simulink subsystem "Environment"  (R2025b)
settings: Solver=VariableStepAuto  StartTime=0.0  StopTime=10.0  RelTol=1e-3
undefined symbols (not defined in the file): ln, Newton, Raphson, SimIn, SimPar
libraries: simulink x7, libAxisTransformations x1
settings Model: Creator=tbritton  LastModifiedBy=bullo
settings SolverCC: AlgebraicLoopSolver=TrustRegion
settings OptimizationCC: ReuseModelBlockBuffer=off
settings DebuggingCC: UnconnectedInputMsg=warning  UnconnectedOutputMsg=warning  UnconnectedLineMsg=warning
settings ModelReferenceCC: EnableRefExpFcnMdlSchedulingChecks=on
settings RTWCC: GPUComputeCapability=3.5  DLArmComputeVersion=19.05

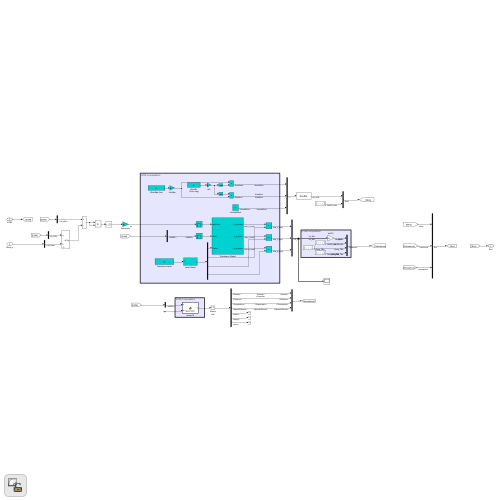
[thumbnail: Simulink's stored preview of the top-level diagram]
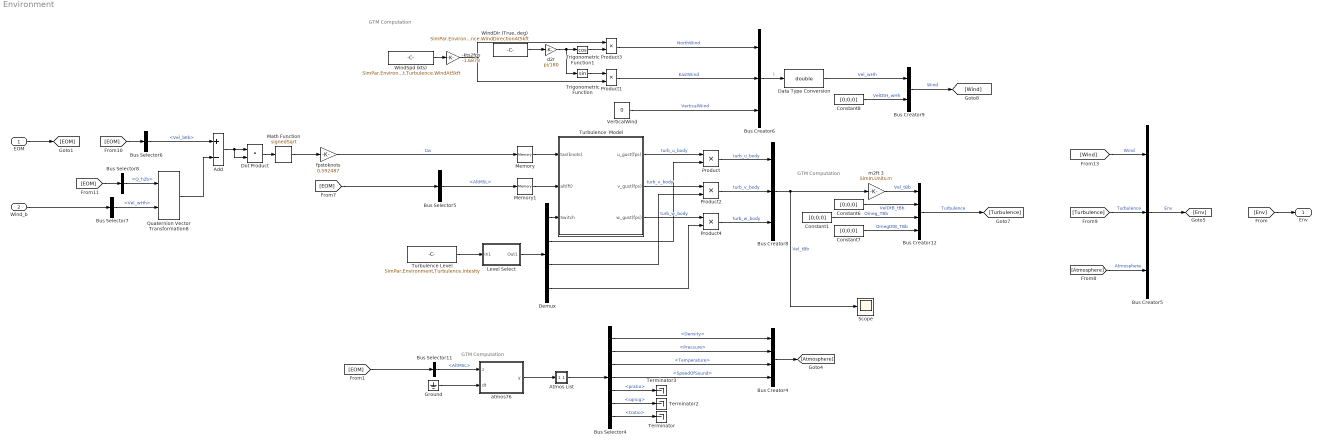
== system Environment ==
  note: GTM Computation
  note: GTM Computation
  note: GTM Computation
  EOM : Inport  OutDataTypeStr=Bus: EomBus
  Wind_b : Inport  Port=2
  -kts2fps : Gain  Gain=-1.6878  SaturateOnIntegerOverflow=on  OutDataTypeStr=Inherit: Same as input  ParamDataTypeStr=Inherit: Same as input
  Add : Sum  Inputs=+-
  Atmos List : Subsystem
  Bus Creator12 : BusCreator  Inputs=4  OutDataTypeStr=Bus: TurbulenceBus
  Bus Creator4 : BusCreator  Inputs=4
  Bus Creator5 : BusCreator  Inputs=3  OutDataTypeStr=Bus: EnvironmentBus
  Bus Creator6 : BusCreator  Inputs=3
  Bus Creator8 : BusCreator  Inputs=3
  Bus Creator9 : BusCreator  Inputs=2  OutDataTypeStr=Bus: WindBus
  Bus Selector11 : BusSelector  OutputSignals=WorldRelativeData.AltMSL
  Bus Selector4 : BusSelector  OutputSignals=Density,Pressure,Temperature,SpeedOfSound,pratio,sqrsig,tratio
  Bus Selector5 : BusSelector  OutputSignals=WorldRelativeData.AltMSL
  Bus Selector6 : BusSelector  OutputSignals=WorldRelativeData.Vel_bEb
  Bus Selector7 : BusSelector  OutputSignals=Wind.Vel_wHh
  Bus Selector8 : BusSelector  OutputSignals=WorldRelativeData.Q_h2b
  Constant{1,6..8} (4 alike) : Constant  Value=[0;0;0]
  Data Type Conversion : DataTypeConversion  OutDataTypeStr=double  SaturateOnIntegerOverflow=off  RndMeth=Floor
  Demux : Demux
  Dot Product : DotProduct  OutDataTypeStr=Inherit: Inherit via internal rule
  Ground : Ground
  Level Select : Subsystem
  Math Function : Sqrt  Operator=signedSqrt  AlgorithmType=Newton-Raphson
  Memory : Memory  InitialCondition=70
  Memory1 : Memory  InitialCondition=1000
  Product : Product  RndMeth=Zero
  Product1 : Product  Inputs=**  InputSameDT=on  SaturateOnIntegerOverflow=on  OutDataTypeStr=Inherit: Same as first input
  Product2 : Product  RndMeth=Zero
  Product3 : Product  Inputs=**  InputSameDT=on  SaturateOnIntegerOverflow=on  OutDataTypeStr=Inherit: Same as first input
  Product4 : Product  RndMeth=Zero
  Quaternion Vector Transformation8 : libAxisTransformations/Quaternion Vector Transformation  n=0
  Scope : Scope
      settings: DataLoggingVariableName=ScopeData16
  Terminator : Terminator
  Terminator2 : Terminator
  Terminator3 : Terminator
  Trigonometric Function : Trigonometry
  Trigonometric Function1 : Trigonometry  Operator=cos
  Turbulence  Model : Subsystem
  Turbulence Level : Constant  Value=SimPar.Environment.Turbulence.intesity
  VerticalWind : Constant  Value=0
  "WindDir (True, deg)" : Constant  Value=SimPar.Environment.Turbulence.WindDirectionAt5kft
  WindSpd (kts) : Constant  Value=SimPar.Environment.Turbulence.WindAt5kft
  atmos76 : MATLAB Function  TreatAsAtomicUnit=on
  d2r : Gain  Gain=pi/180  SaturateOnIntegerOverflow=on  OutDataTypeStr=Inherit: Same as input  ParamDataTypeStr=Inherit: Same as input
  fpstoknots : Gain  Gain=0.592487
  m2ft 3 : Gain  Gain=SimIn.Units.m
  Env : Outport  OutDataTypeStr=Bus: EnvironmentBus  VectorParamsAs1DForOutWhenUnconnected=off
  wires:
  Data Type Conversion/1 -> Bus Creator9/1  "Vel_wHh"
  [EOM] -> Bus Selector8/1
  [EOM] -> Bus Selector6/1
  Quaternion Vector Transformation8/1 -> Add/2
  fpstoknots/1 -> Memory/1  "tas"
  Math Function/1 -> fpstoknots/1
  Wind_b/1 -> Bus Selector7/1
  Add/1 -> Dot Product/1, Dot Product/2
  Dot Product/1 -> Math Function/1
  Bus Creator12/1 -> [Turbulence]  "Turbulence"
  Constant7/1 -> Bus Creator12/4  "OmegDtB_TBb"
  Constant6/1 -> Bus Creator12/2  "VelDtB_tBb"
  m2ft 3/1 -> Bus Creator12/1  "Vel_tBb"
  Constant1/1 -> Bus Creator12/3  "Omeg_TBb"
  [EOM] -> Bus Selector11/1
  Ground/1 -> atmos76/2(dt)
  Bus Selector11/1 -> atmos76/1(z)  "<AltMSL>"
  atmos76/1(y) -> Atmos List/1(I)
  Turbulence  Model/3(w_gust(fps)) -> Product4/1  "turb_w_body"
  Memory/1 -> Turbulence  Model/1(tas(knots))
  Level Select/1(Out1) -> Demux/1
  Turbulence  Model/1(u_gust(fps)) -> Product/1  "turb_u_body"
  Turbulence Level/1 -> Level Select/1(In1)
  Trigonometric Function/1 -> Product1/1
  Turbulence  Model/2(v_gust(fps)) -> Product2/1  "turb_v_body"
  "WindDir (True, deg)"/1 -> d2r/1
  d2r/1 -> Trigonometric Function/1, Trigonometric Function1/1
  Demux/1 -> Turbulence  Model/3(Switch)
  Demux/2 -> Product/2
  -kts2fps/1 -> Product3/1, Product1/2
  Demux/4 -> Product4/2
  Demux/3 -> Product2/2
  WindSpd (kts)/1 -> -kts2fps/1
  Trigonometric Function1/1 -> Product3/2
  Memory1/1 -> Turbulence  Model/2(alt(ft))
  [EOM] -> Bus Selector5/1
  Bus Selector5/1 -> Memory1/1  "<AltMSL>"
  [Turbulence] -> Bus Creator5/2  "Turbulence"
  [Wind] -> Bus Creator5/1  "Wind"
  [Atmosphere] -> Bus Creator5/3  "Atmosphere"
  Bus Creator5/1 -> [Env]  "Env"
  Bus Selector4/7 -> Terminator/1  "<tratio>"
  Bus Selector4/6 -> Terminator2/1  "<sqrsig>"
  Bus Selector4/5 -> Terminator3/1  "<pratio>"
  Atmos List/1(O) -> Bus Selector4/1
  [Env] -> Env/1
  EOM/1 -> [EOM]
  Bus Creator4/1 -> [Atmosphere]
  Bus Selector4/3 -> Bus Creator4/3  "<Temperature>"
  Bus Selector4/1 -> Bus Creator4/1  "<Density>"
  Bus Selector4/4 -> Bus Creator4/4  "<SpeedOfSound>"
  Bus Selector4/2 -> Bus Creator4/2  "<Pressure>"
  Product/1 -> Bus Creator8/1  "turb_u_body"
  Product2/1 -> Bus Creator8/2  "turb_v_body"
  Product4/1 -> Bus Creator8/3  "turb_w_body"
  Bus Selector6/1 -> Add/1  "<Vel_bEb>"
  Bus Selector8/1 -> Quaternion Vector Transformation8/1  "<Q_h2b>"
  Bus Selector7/1 -> Quaternion Vector Transformation8/2  "<Vel_wHh>"
  Constant8/1 -> Bus Creator9/2  "VelDtH_wHh"
  Product3/1 -> Bus Creator6/1  "NorthWind"
  Product1/1 -> Bus Creator6/2  "EastWind"
  Bus Creator9/1 -> [Wind]  "Wind"
  VerticalWind/1 -> Bus Creator6/3  "VerticalWind"
  Bus Creator6/1 -> Data Type Conversion/1  "l"
  Bus Creator8/1 -> Scope/1, m2ft 3/1  "Vel_tBb"

== system Environment/Atmos List ==
  I : Inport
  BusCreator : BusCreator  Inputs=7
  Demux2 : Demux  Outputs=6
      settings: DisplayOption=none
  Divide : Product  Inputs=*/
  Standard Temp. K : Constant  Value=288.15
  O : Outport  VectorParamsAs1DForOutWhenUnconnected=off
  wires:
  Demux2/6 -> BusCreator/6  "sqrsig"
  Demux2/5 -> BusCreator/5  "pratio"
  Demux2/4 -> BusCreator/4  "SpeedOfSound"
  Demux2/3 -> BusCreator/3, Divide/1  "Temperature"
  Demux2/2 -> BusCreator/2  "Pressure"
  Demux2/1 -> BusCreator/1  "Density"
  I/1 -> Demux2/1
  BusCreator/1 -> O/1
  Standard Temp. K/1 -> Divide/2
  Divide/1 -> BusCreator/7  "tratio"

== system Environment/Level Select ==
  In1 : Inport
  Light : Constant  Value=[1 0.2 0.2 0.17]
  Moderate : Constant  Value=[1 0.4 0.4 0.34]
  Multiport Switch : MultiPortSwitch  Inputs=4  SaturateOnIntegerOverflow=off  InputSameDT=off
  Severe : Constant  Value=[1 0.4 1.152 0.34]
  Turbulence Off : Constant  Value=[0 0 0 0]
  Out1 : Outport
  wires:
  In1/1 -> Multiport Switch/1
  Turbulence Off/1 -> Multiport Switch/2
  Light/1 -> Multiport Switch/3
  Moderate/1 -> Multiport Switch/4
  Severe/1 -> Multiport Switch/5
  Multiport Switch/1 -> Out1/1

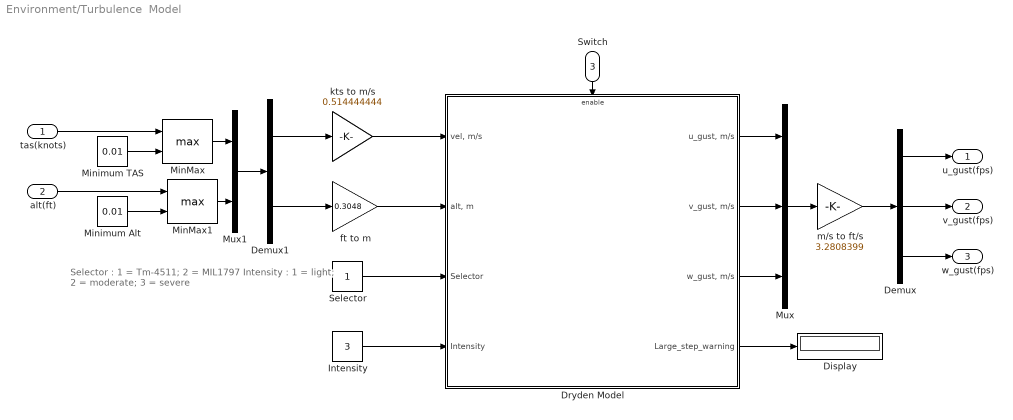
== system Environment/Turbulence  Model ==
  note: Selector :  1 = Tm-4511;  2 = MIL1797
      |             Intensity :  1 = light;  2 = moderate;  3 = severe
  tas(knots) : Inport
  alt(ft) : Inport  Port=2
  Switch : Inport  Port=3
  Demux : Demux  Outputs=3
  Demux1 : Demux  Outputs=2
  Display : Display
  Dryden Model : Subsystem  mask{longseed=3366+521, latseed=23+521, vertseed=1369+521, dt=SimIn.Environment.Turbulence.dT, Step_warning_pct=.11}
      mask prompts: longseed "Longitudinal Random Number Seed"; latseed "Lateral Random Number Seed"; vertseed "Vertical Random Number Seed"; dt "Turbulence model time step, sec"; Step_warning_pct "Threshhold for stepsize warning (%)"
  Intensity : Constant  Value=3
  MinMax : MinMax  Function=max  Inputs=2
  MinMax1 : MinMax  Function=max  Inputs=2
  Minimum Alt : Constant  Value=0.01
  Minimum TAS : Constant  Value=0.01
  Mux : Mux  Inputs=3
  Mux1 : Mux  Inputs=2
  Selector : Constant
  ft to m : Gain  Gain=0.3048
  kts to m/s : Gain  Gain=0.514444444
  m/s to ft/s : Gain  Gain=3.2808399
  u_gust(fps) : Outport
  v_gust(fps) : Outport  Port=2
  w_gust(fps) : Outport  Port=3
  wires:
  Switch/1 -> Dryden Model/Enable
  Dryden Model/1("u_gust, m/s") -> Mux/1
  Dryden Model/2("v_gust, m/s") -> Mux/2
  Dryden Model/3("w_gust, m/s") -> Mux/3
  Demux/3 -> w_gust(fps)/1
  Demux/2 -> v_gust(fps)/1
  Demux/1 -> u_gust(fps)/1
  Dryden Model/4(Large_step_warning) -> Display/1
  Mux/1 -> m/s to ft/s/1
  m/s to ft/s/1 -> Demux/1
  MinMax1/1 -> Mux1/2
  MinMax/1 -> Mux1/1
  alt(ft)/1 -> MinMax1/1
  Minimum Alt/1 -> MinMax1/2
  Minimum TAS/1 -> MinMax/2
  tas(knots)/1 -> MinMax/1
  Mux1/1 -> Demux1/1
  Demux1/2 -> ft to m/1
  Demux1/1 -> kts to m/s/1
  Intensity/1 -> Dryden Model/4(Intensity)
  Selector/1 -> Dryden Model/3(Selector)
  ft to m/1 -> Dryden Model/2("alt, m")
  kts to m/s/1 -> Dryden Model/1("vel, m/s")

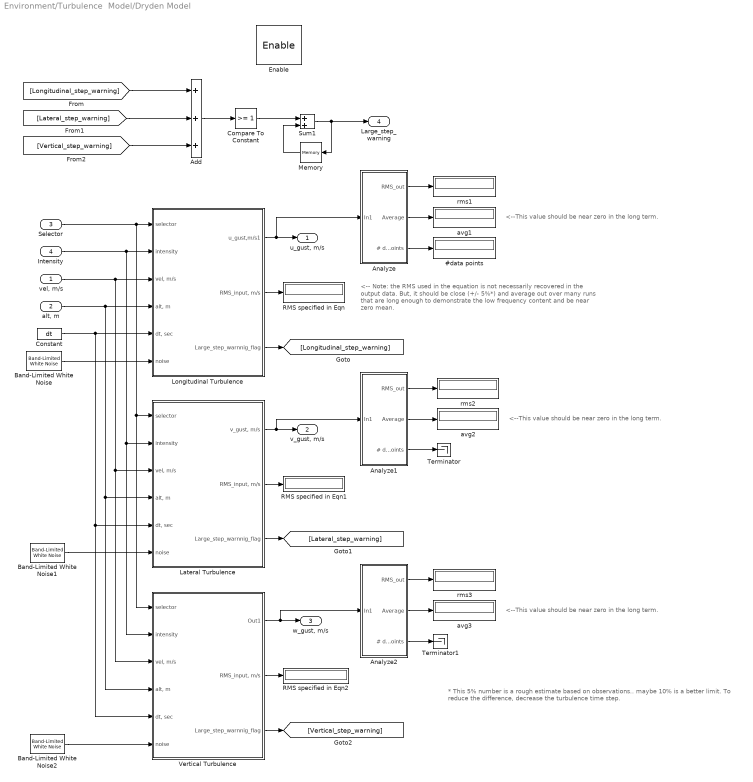
== system Environment/Turbulence  Model/Dryden Model ==
  note: * This 5% number is a rough estimate based on observations.. maybe 10% is a better limit.
      | To reduce the difference, decrease the turbulence time step.
  note: <--This value should be near zero in the long term.
  note: <--This value should be near zero in the long term.
  note: <--This value should be near zero in the long term.
  note: <-- Note: the RMS used in the equation is not necessarily recovered
      | in the output data.  But, it should be close (+/- 5%*) and  average out over
      | many runs that are long enough to demonstrate the low frequency
      | content and be near zero mean.
  "vel, m/s" : Inport
  "alt, m" : Inport  Port=2
  Selector : Inport  Port=3
  Intensity : Inport  Port=4
  Enable : EnablePort  StatesWhenEnabling=reset
  #data points : Display
  Add : Sum  Inputs=3
  Analyze : Subsystem
  Analyze1 : Subsystem
  Analyze2 : Subsystem
  Band-Limited White Noise : simulink/Sources/Band-Limited White Noise  Cov=dt  Ts=dt  seed=longseed
  Band-Limited White Noise1 : simulink/Sources/Band-Limited White Noise  Cov=dt  Ts=dt  seed=latseed
  Band-Limited White Noise2 : simulink/Sources/Band-Limited White Noise  Cov=dt  Ts=dt  seed=vertseed
  Compare To Constant : simulink/Logic and Bit Operations/Compare To Constant  relop=>=  const=1  OutDataTypeStr=uint8  ZeroCross=off
  Constant : Constant  Value=dt
  Lateral Turbulence : Subsystem
  Longitudinal Turbulence : Subsystem
  Memory : Memory
  RMS specified in Eqn : Display
  RMS specified in Eqn1 : Display
  RMS specified in Eqn2 : Display
  Sum1 : Sum  Inputs=2  SaturateOnIntegerOverflow=on
  Terminator : Terminator
  Terminator1 : Terminator
  Vertical Turbulence : Subsystem
  avg1 : Display
  avg2 : Display
  avg3 : Display
  rms1 : Display
  rms2 : Display
  rms3 : Display
  "u_gust, m/s" : Outport  OutputWhenDisabled=reset  InitialOutput=0
  "v_gust, m/s" : Outport  Port=2  OutputWhenDisabled=reset  InitialOutput=0
  "w_gust, m/s" : Outport  Port=3  OutputWhenDisabled=reset  InitialOutput=0
  Large_step_warning : Outport  Port=4  OutputWhenDisabled=reset  InitialOutput=0
  wires:
  Sum1/1 -> Memory/1, Large_step_warning/1
  Memory/1 -> Sum1/2
  Compare To Constant/1 -> Sum1/1
  Vertical Turbulence/3(Large_step_warnnig_flag) -> [Vertical_step_warning]
  Lateral Turbulence/3(Large_step_warnnig_flag) -> [Lateral_step_warning]
  Longitudinal Turbulence/3(Large_step_warnnig_flag) -> [Longitudinal_step_warning]
  [Lateral_step_warning] -> Add/2
  [Vertical_step_warning] -> Add/3
  [Longitudinal_step_warning] -> Add/1
  Add/1 -> Compare To Constant/1
  Band-Limited White Noise/1 -> Longitudinal Turbulence/6(noise)
  Analyze2/3(# data points) -> Terminator1/1
  Analyze1/3(# data points) -> Terminator/1
  Analyze/3(# data points) -> #data points/1
  Vertical Turbulence/2("RMS_input, m/s") -> RMS specified in Eqn2/1
  Lateral Turbulence/2("RMS_input, m/s") -> RMS specified in Eqn1/1
  Longitudinal Turbulence/2("RMS_input, m/s") -> RMS specified in Eqn/1
  Analyze2/2(Average) -> avg3/1
  Analyze2/1(RMS_out) -> rms3/1
  Vertical Turbulence/1(Out1) -> Analyze2/1(In1), "w_gust, m/s"/1
  Analyze1/2(Average) -> avg2/1
  Analyze1/1(RMS_out) -> rms2/1
  Lateral Turbulence/1("v_gust, m/s") -> Analyze1/1(In1), "v_gust, m/s"/1
  Analyze/2(Average) -> avg1/1
  Longitudinal Turbulence/1(u_gust,m/s1) -> Analyze/1(In1), "u_gust, m/s"/1
  Analyze/1(RMS_out) -> rms1/1
  Intensity/1 -> Lateral Turbulence/2(intensity), Vertical Turbulence/2(intensity), Longitudinal Turbulence/2(intensity)
  Band-Limited White Noise2/1 -> Vertical Turbulence/6(noise)
  Selector/1 -> Lateral Turbulence/1(selector), Vertical Turbulence/1(selector), Longitudinal Turbulence/1(selector)
  Band-Limited White Noise1/1 -> Lateral Turbulence/6(noise)
  Constant/1 -> Lateral Turbulence/5("dt, sec"), Vertical Turbulence/5("dt, sec"), Longitudinal Turbulence/5("dt, sec")
  "alt, m"/1 -> Lateral Turbulence/4("alt, m"), Vertical Turbulence/4("alt, m"), Longitudinal Turbulence/4("alt, m")
  "vel, m/s"/1 -> Lateral Turbulence/3("vel, m/s"), Vertical Turbulence/3("vel, m/s"), Longitudinal Turbulence/3("vel, m/s")

== system Environment/Turbulence  Model/Dryden Model/Analyze ==
  In1 : Inport
  Constant1 : Constant
  Constant3 : Constant  Value=0
  Constant5 : Constant  Value=dt
  Digital Clock1 : DigitalClock  SampleTime=dt
  Fcn : Fcn  Expr=sqrt(u)
  Memory : Memory
  Memory1 : Memory
  MinMax : MinMax  Function=max  Inputs=2
  Product : Product  SaturateOnIntegerOverflow=on  OutDataTypeStr=Inherit: Same as first input
  Product2 : Product  Inputs=/*  SaturateOnIntegerOverflow=on  OutDataTypeStr=Inherit: Same as first input
  Product3 : Product  Inputs=/*  SaturateOnIntegerOverflow=on  OutDataTypeStr=Inherit: Same as first input
  Product4 : Product  Inputs=/*  SaturateOnIntegerOverflow=on  OutDataTypeStr=Inherit: Same as first input
  Sum : Sum  Inputs=++-  SaturateOnIntegerOverflow=on
  Sum1 : Sum  Inputs=2  SaturateOnIntegerOverflow=on
  RMS_out : Outport
  Average : Outport  Port=2
  # data points : Outport  Port=3
  wires:
  MinMax/1 -> Product2/1, Product4/1
  Constant1/1 -> MinMax/2
  In1/1 -> Sum1/1, Product/1, Product/2
  Product/1 -> Sum/2
  Sum/1 -> Memory1/1, Product2/2
  Sum1/1 -> Memory/1, Product4/2
  Product2/1 -> Fcn/1
  Memory/1 -> Sum1/2
  Memory1/1 -> Sum/1
  Constant3/1 -> Sum/3
  Constant5/1 -> Product3/1
  Digital Clock1/1 -> Product3/2
  Product3/1 -> MinMax/1, # data points/1
  Fcn/1 -> RMS_out/1
  Product4/1 -> Average/1

== system Environment/Turbulence  Model/Dryden Model/Analyze1 ==
  In1 : Inport
  Constant1 : Constant
  Constant3 : Constant  Value=0
  Constant5 : Constant  Value=dt
  Digital Clock1 : DigitalClock  SampleTime=dt
  Fcn : Fcn  Expr=sqrt(u)
  Memory : Memory
  Memory1 : Memory
  MinMax : MinMax  Function=max  Inputs=2
  Product : Product  SaturateOnIntegerOverflow=on  OutDataTypeStr=Inherit: Same as first input
  Product2 : Product  Inputs=/*  SaturateOnIntegerOverflow=on  OutDataTypeStr=Inherit: Same as first input
  Product3 : Product  Inputs=/*  SaturateOnIntegerOverflow=on  OutDataTypeStr=Inherit: Same as first input
  Product4 : Product  Inputs=/*  SaturateOnIntegerOverflow=on  OutDataTypeStr=Inherit: Same as first input
  Sum : Sum  Inputs=++-  SaturateOnIntegerOverflow=on
  Sum1 : Sum  Inputs=2  SaturateOnIntegerOverflow=on
  RMS_out : Outport
  Average : Outport  Port=2
  # data points : Outport  Port=3
  wires:
  Product4/1 -> Average/1
  Fcn/1 -> RMS_out/1
  Product3/1 -> # data points/1, MinMax/1
  Digital Clock1/1 -> Product3/2
  Constant5/1 -> Product3/1
  Constant3/1 -> Sum/3
  Memory1/1 -> Sum/1
  Memory/1 -> Sum1/2
  Product2/1 -> Fcn/1
  Sum1/1 -> Product4/2, Memory/1
  Sum/1 -> Product2/2, Memory1/1
  Product/1 -> Sum/2
  In1/1 -> Product/2, Product/1, Sum1/1
  Constant1/1 -> MinMax/2
  MinMax/1 -> Product4/1, Product2/1

== system Environment/Turbulence  Model/Dryden Model/Analyze2 ==
  In1 : Inport
  Constant1 : Constant
  Constant3 : Constant  Value=0
  Constant5 : Constant  Value=dt
  Digital Clock1 : DigitalClock  SampleTime=dt
  Fcn : Fcn  Expr=sqrt(u)
  Memory : Memory
  Memory1 : Memory
  MinMax : MinMax  Function=max  Inputs=2
  Product : Product  SaturateOnIntegerOverflow=on  OutDataTypeStr=Inherit: Same as first input
  Product2 : Product  Inputs=/*  SaturateOnIntegerOverflow=on  OutDataTypeStr=Inherit: Same as first input
  Product3 : Product  Inputs=/*  SaturateOnIntegerOverflow=on  OutDataTypeStr=Inherit: Same as first input
  Product4 : Product  Inputs=/*  SaturateOnIntegerOverflow=on  OutDataTypeStr=Inherit: Same as first input
  Sum : Sum  Inputs=++-  SaturateOnIntegerOverflow=on
  Sum1 : Sum  Inputs=2  SaturateOnIntegerOverflow=on
  RMS_out : Outport
  Average : Outport  Port=2
  # data points : Outport  Port=3
  wires:
  MinMax/1 -> Product2/1, Product4/1
  Constant1/1 -> MinMax/2
  In1/1 -> Sum1/1, Product/1, Product/2
  Product/1 -> Sum/2
  Sum/1 -> Memory1/1, Product2/2
  Sum1/1 -> Memory/1, Product4/2
  Product2/1 -> Fcn/1
  Memory/1 -> Sum1/2
  Memory1/1 -> Sum/1
  Constant3/1 -> Sum/3
  Constant5/1 -> Product3/1
  Digital Clock1/1 -> Product3/2
  Product3/1 -> MinMax/1, # data points/1
  Fcn/1 -> RMS_out/1
  Product4/1 -> Average/1

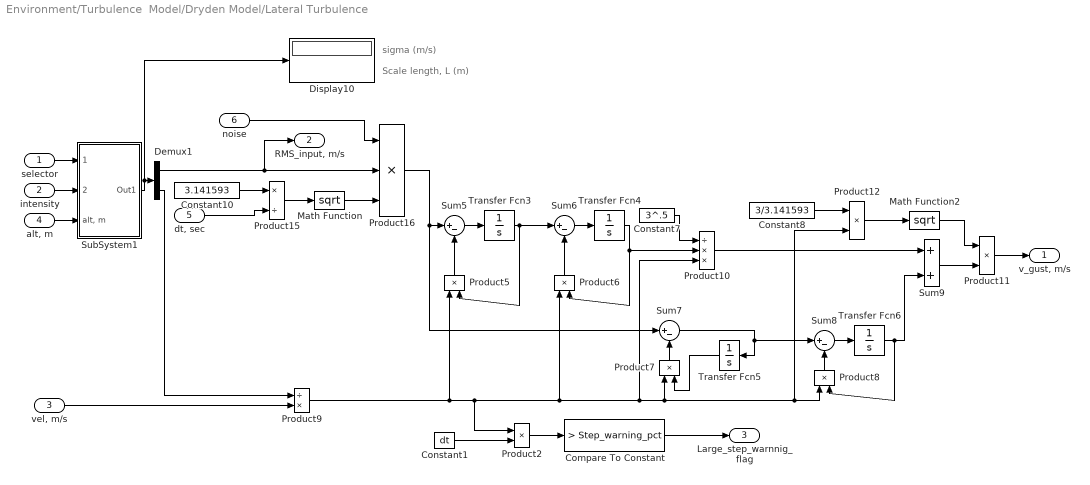
== system Environment/Turbulence  Model/Dryden Model/Lateral Turbulence ==
  note: Scale length, L (m)
  note: sigma (m/s)
  selector : Inport
  intensity : Inport  Port=2
  "vel, m/s" : Inport  Port=3
  "alt, m" : Inport  Port=4
  "dt, sec" : Inport  Port=5
  noise : Inport  Port=6
  Compare To Constant : simulink/Logic and Bit Operations/Compare To Constant  relop=>  const=Step_warning_pct  OutDataTypeStr=uint8  ZeroCross=off
  Constant1 : Constant  Value=dt
  Constant10 : Constant  Value=3.141593
  Constant7 : Constant  Value=3^.5
  Constant8 : Constant  Value=3/3.141593
  Demux1 : Demux  Outputs=2
      settings: DisplayOption=none
  Display10 : Display
  Math Function : Math  Operator=sqrt  SignedPower=on
  Math Function2 : Math  Operator=sqrt  SignedPower=on
  Product10 : Product  Inputs=/**  InputSameDT=on  SaturateOnIntegerOverflow=on  OutDataTypeStr=Inherit: Same as first input
  Product11 : Product  Inputs=**  InputSameDT=on  SaturateOnIntegerOverflow=on  OutDataTypeStr=Inherit: Same as first input
  Product12 : Product  Inputs=**  InputSameDT=on  SaturateOnIntegerOverflow=on  OutDataTypeStr=Inherit: Same as first input
  Product15 : Product  Inputs=*/  InputSameDT=on  SaturateOnIntegerOverflow=on  OutDataTypeStr=Inherit: Same as first input
  Product16 : Product  Inputs=***  InputSameDT=on  SaturateOnIntegerOverflow=on  OutDataTypeStr=Inherit: Same as first input
  Product{2,5..8} (5 alike) : Product  InputSameDT=on  SaturateOnIntegerOverflow=on  OutDataTypeStr=Inherit: Same as first input
  Product9 : Product  Inputs=/*  InputSameDT=on  SaturateOnIntegerOverflow=on  OutDataTypeStr=Inherit: Same as first input
  SubSystem1 : Subsystem
  Sum{5..8} (4 alike) : Sum  Inputs=|+-  InputSameDT=on  SaturateOnIntegerOverflow=on  OutDataTypeStr=Inherit: Same as first input
  Sum9 : Sum  Inputs=2  InputSameDT=on  SaturateOnIntegerOverflow=on  OutDataTypeStr=Inherit: Same as first input
  Transfer Fcn{3..6} (4 alike) : TransferFcn  Numerator=1  Denominator=[1 0]
  "v_gust, m/s" : Outport
  "RMS_input, m/s" : Outport  Port=2
  Large_step_warnnig_flag : Outport  Port=3
  wires:
  Compare To Constant/1 -> Large_step_warnnig_flag/1
  Product2/1 -> Compare To Constant/1
  Constant1/1 -> Product2/2
  Math Function/1 -> Product16/3
  intensity/1 -> SubSystem1/2(intensity)
  selector/1 -> SubSystem1/1(selector)
  "alt, m"/1 -> SubSystem1/3("alt, m")
  Demux1/2 -> Product9/1
  SubSystem1/1(Out1) -> Display10/1, Demux1/1
  Product16/1 -> Sum7/1, Sum5/1
  Demux1/1 -> Product16/2, "RMS_input, m/s"/1
  "dt, sec"/1 -> Product15/2
  Product9/1 -> Product2/1, Product10/3, Product12/2, Product8/1, Product7/1, Product6/1, Product5/1
  "vel, m/s"/1 -> Product9/2
  Product12/1 -> Math Function2/1
  Constant8/1 -> Product12/1
  Math Function2/1 -> Product11/1
  Sum9/1 -> Product11/2
  Constant7/1 -> Product10/1
  Product10/1 -> Sum9/1
  Transfer Fcn6/1 -> Sum9/2, Product8/2
  Sum7/1 -> Sum8/1, Transfer Fcn5/1
  Product8/1 -> Sum8/2
  Sum8/1 -> Transfer Fcn6/1
  Product7/1 -> Sum7/2
  Transfer Fcn5/1 -> Product7/2
  Transfer Fcn4/1 -> Product10/2, Product6/2
  Transfer Fcn3/1 -> Sum6/1, Product5/2
  Product6/1 -> Sum6/2
  Sum6/1 -> Transfer Fcn4/1
  Sum5/1 -> Transfer Fcn3/1
  Product5/1 -> Sum5/2
  noise/1 -> Product16/1
  Constant10/1 -> Product15/1
  Product15/1 -> Math Function/1
  Product11/1 -> "v_gust, m/s"/1

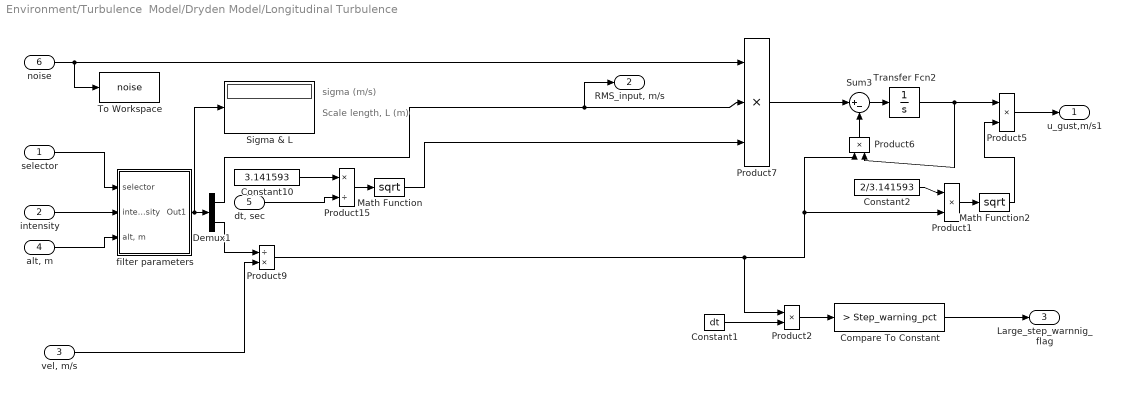
== system Environment/Turbulence  Model/Dryden Model/Longitudinal Turbulence ==
  note: Scale length, L (m)
  note: sigma (m/s)
  selector : Inport
  intensity : Inport  Port=2
  "vel, m/s" : Inport  Port=3
  "alt, m" : Inport  Port=4
  "dt, sec" : Inport  Port=5
  noise : Inport  Port=6
  Compare To Constant : simulink/Logic and Bit Operations/Compare To Constant  relop=>  const=Step_warning_pct  OutDataTypeStr=uint8  ZeroCross=off
  Constant1 : Constant  Value=dt
  Constant10 : Constant  Value=3.141593
  Constant2 : Constant  Value=2/3.141593
  Demux1 : Demux  Outputs=2
      settings: DisplayOption=none
  Math Function : Math  Operator=sqrt  SignedPower=on
  Math Function2 : Math  Operator=sqrt  SignedPower=on
  Product1 : Product  Inputs=**  InputSameDT=on  SaturateOnIntegerOverflow=on  OutDataTypeStr=Inherit: Same as first input
  Product15 : Product  Inputs=*/  InputSameDT=on  SaturateOnIntegerOverflow=on  OutDataTypeStr=Inherit: Same as first input
  Product2 : Product  InputSameDT=on  SaturateOnIntegerOverflow=on  OutDataTypeStr=Inherit: Same as first input
  Product5 : Product  Inputs=**  InputSameDT=on  SaturateOnIntegerOverflow=on  OutDataTypeStr=Inherit: Same as first input
  Product6 : Product  InputSameDT=on  SaturateOnIntegerOverflow=on  OutDataTypeStr=Inherit: Same as first input
  Product7 : Product  Inputs=***  InputSameDT=on  SaturateOnIntegerOverflow=on  OutDataTypeStr=Inherit: Same as first input
  Product9 : Product  Inputs=/*  InputSameDT=on  SaturateOnIntegerOverflow=on  OutDataTypeStr=Inherit: Same as first input
  Sigma & L : Display
  Sum3 : Sum  Inputs=|+-  InputSameDT=on  SaturateOnIntegerOverflow=on  OutDataTypeStr=Inherit: Same as first input
  To Workspace : ToWorkspace  VariableName=noise  SampleTime=-1
  Transfer Fcn2 : TransferFcn  Numerator=1  Denominator=[1 0]
  filter parameters : Subsystem
  u_gust,m/s1 : Outport
  "RMS_input, m/s" : Outport  Port=2
  Large_step_warnnig_flag : Outport  Port=3
  wires:
  Compare To Constant/1 -> Large_step_warnnig_flag/1
  Product2/1 -> Compare To Constant/1
  Constant1/1 -> Product2/2
  Product7/1 -> Sum3/1
  Product6/1 -> Sum3/2
  Product5/1 -> u_gust,m/s1/1
  Math Function2/1 -> Product5/2
  Product1/1 -> Math Function2/1
  Constant2/1 -> Product1/1
  Sum3/1 -> Transfer Fcn2/1
  Transfer Fcn2/1 -> Product5/1, Product6/2
  intensity/1 -> filter parameters/2(intensity)
  Demux1/1 -> "RMS_input, m/s"/1, Product7/2
  Demux1/2 -> Product9/1
  filter parameters/1(Out1) -> Demux1/1, Sigma & L/1
  noise/1 -> Product7/1, To Workspace/1
  "dt, sec"/1 -> Product15/2
  "vel, m/s"/1 -> Product9/2
  Constant10/1 -> Product15/1
  Product9/1 -> Product2/1, Product1/2, Product6/1
  Math Function/1 -> Product7/3
  Product15/1 -> Math Function/1
  selector/1 -> filter parameters/1(selector)
  "alt, m"/1 -> filter parameters/3("alt, m")

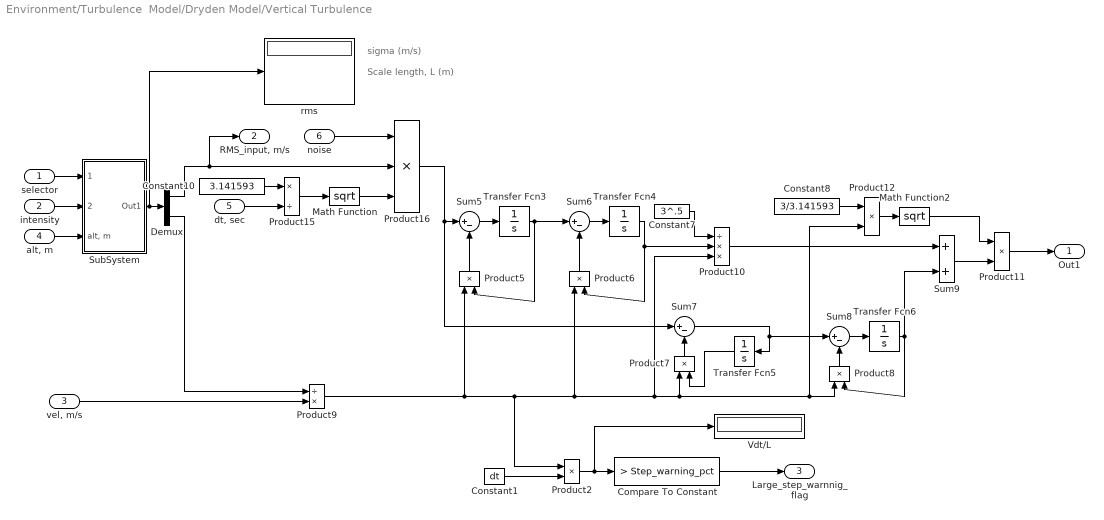
== system Environment/Turbulence  Model/Dryden Model/Vertical Turbulence ==
  note: Scale length, L (m)
  note: sigma (m/s)
  selector : Inport
  intensity : Inport  Port=2
  "vel, m/s" : Inport  Port=3
  "alt, m" : Inport  Port=4
  "dt, sec" : Inport  Port=5
  noise : Inport  Port=6
  Compare To Constant : simulink/Logic and Bit Operations/Compare To Constant  relop=>  const=Step_warning_pct  OutDataTypeStr=uint8  ZeroCross=off
  Constant1 : Constant  Value=dt
  Constant10 : Constant  Value=3.141593
  Constant7 : Constant  Value=3^.5
  Constant8 : Constant  Value=3/3.141593
  Demux : Demux  Outputs=2
      settings: DisplayOption=none
  Math Function : Math  Operator=sqrt  SignedPower=on
  Math Function2 : Math  Operator=sqrt  SignedPower=on
  Product10 : Product  Inputs=/**  InputSameDT=on  SaturateOnIntegerOverflow=on  OutDataTypeStr=Inherit: Same as first input
  Product11 : Product  Inputs=**  InputSameDT=on  SaturateOnIntegerOverflow=on  OutDataTypeStr=Inherit: Same as first input
  Product12 : Product  Inputs=**  InputSameDT=on  SaturateOnIntegerOverflow=on  OutDataTypeStr=Inherit: Same as first input
  Product15 : Product  Inputs=*/  InputSameDT=on  SaturateOnIntegerOverflow=on  OutDataTypeStr=Inherit: Same as first input
  Product16 : Product  Inputs=***  InputSameDT=on  SaturateOnIntegerOverflow=on  OutDataTypeStr=Inherit: Same as first input
  Product{2,5..8} (5 alike) : Product  InputSameDT=on  SaturateOnIntegerOverflow=on  OutDataTypeStr=Inherit: Same as first input
  Product9 : Product  Inputs=/*  InputSameDT=on  SaturateOnIntegerOverflow=on  OutDataTypeStr=Inherit: Same as first input
  SubSystem : Subsystem
  Sum{5..8} (4 alike) : Sum  Inputs=|+-  InputSameDT=on  SaturateOnIntegerOverflow=on  OutDataTypeStr=Inherit: Same as first input
  Sum9 : Sum  Inputs=2  InputSameDT=on  SaturateOnIntegerOverflow=on  OutDataTypeStr=Inherit: Same as first input
  Transfer Fcn{3..6} (4 alike) : TransferFcn  Numerator=1  Denominator=[1 0]
  Vdt/L : Display
  rms : Display
  Out1 : Outport
  "RMS_input, m/s" : Outport  Port=2
  Large_step_warnnig_flag : Outport  Port=3
  wires:
  Compare To Constant/1 -> Large_step_warnnig_flag/1
  Product2/1 -> Vdt/L/1, Compare To Constant/1
  Constant1/1 -> Product2/2
  intensity/1 -> SubSystem/2("intensity ")
  selector/1 -> SubSystem/1(selector)
  "alt, m"/1 -> SubSystem/3("alt, m")
  SubSystem/1(Out1) -> rms/1, Demux/1
  Demux/2 -> Product9/1
  Demux/1 -> "RMS_input, m/s"/1, Product16/2
  noise/1 -> Product16/1
  Product16/1 -> Sum7/1, Sum5/1
  "dt, sec"/1 -> Product15/2
  Math Function/1 -> Product16/3
  Product9/1 -> Product2/1, Product6/1, Product10/3, Product12/2, Product8/1, Product7/1, Product5/1
  "vel, m/s"/1 -> Product9/2
  Product12/1 -> Math Function2/1
  Constant8/1 -> Product12/1
  Math Function2/1 -> Product11/1
  Sum9/1 -> Product11/2
  Constant7/1 -> Product10/1
  Product10/1 -> Sum9/1
  Transfer Fcn6/1 -> Sum9/2, Product8/2
  Sum7/1 -> Sum8/1, Transfer Fcn5/1
  Product8/1 -> Sum8/2
  Sum8/1 -> Transfer Fcn6/1
  Product7/1 -> Sum7/2
  Transfer Fcn5/1 -> Product7/2
  Transfer Fcn4/1 -> Product10/2, Product6/2
  Transfer Fcn3/1 -> Sum6/1, Product5/2
  Product6/1 -> Sum6/2
  Sum6/1 -> Transfer Fcn4/1
  Sum5/1 -> Transfer Fcn3/1
  Product5/1 -> Sum5/2
  Constant10/1 -> Product15/1
  Product15/1 -> Math Function/1
  Product11/1 -> Out1/1

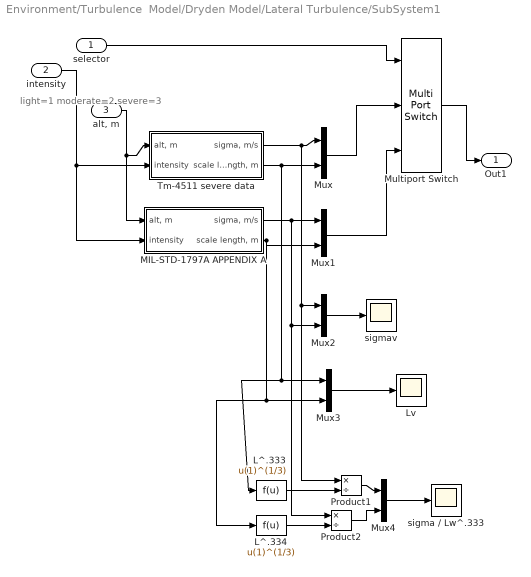
== system Environment/Turbulence  Model/Dryden Model/Lateral Turbulence/SubSystem1 ==
  note: light=1
      | moderate=2
      | severe=3
  selector : Inport
  intensity : Inport  Port=2
  "alt, m" : Inport  Port=3
  L^.333 : Fcn  Expr=u(1)^(1/3)
  L^.334 : Fcn  Expr=u(1)^(1/3)
  Lv : Scope
  "MIL-STD-1797A APPENDIX A " : Subsystem
  Multiport Switch : MultiPortSwitch  Inputs=2
  Mux{,1..4} (5 alike) : Mux  Inputs=2
  Product1 : Product  Inputs=*/  InputSameDT=on  SaturateOnIntegerOverflow=on  OutDataTypeStr=Inherit: Same as first input
  Product2 : Product  Inputs=*/  InputSameDT=on  SaturateOnIntegerOverflow=on  OutDataTypeStr=Inherit: Same as first input
  Tm-4511 severe data : Subsystem
  sigma / Lw^.333 : Scope
  sigmav : Scope
  Out1 : Outport
  wires:
  L^.333/1 -> Product1/2
  Product1/1 -> Mux4/1
  Product2/1 -> Mux4/2
  Mux4/1 -> sigma / Lw^.333/1
  L^.334/1 -> Product2/2
  "MIL-STD-1797A APPENDIX A "/2("scale length, m") -> L^.334/1, Mux3/2, Mux1/2
  Tm-4511 severe data/2("scale length, m") -> L^.333/1, Mux3/1, Mux/2
  "MIL-STD-1797A APPENDIX A "/1("sigma, m/s") -> Product2/1, Mux2/2, Mux1/1
  Mux2/1 -> sigmav/1
  Mux3/1 -> Lv/1
  Mux1/1 -> Multiport Switch/3
  intensity/1 -> Tm-4511 severe data/2(intensity), "MIL-STD-1797A APPENDIX A "/2(intensity)
  "alt, m"/1 -> "MIL-STD-1797A APPENDIX A "/1("alt, m"), Tm-4511 severe data/1("alt, m")
  Mux/1 -> Multiport Switch/2
  Tm-4511 severe data/1("sigma, m/s") -> Product1/1, Mux2/1, Mux/1
  Multiport Switch/1 -> Out1/1
  selector/1 -> Multiport Switch/1

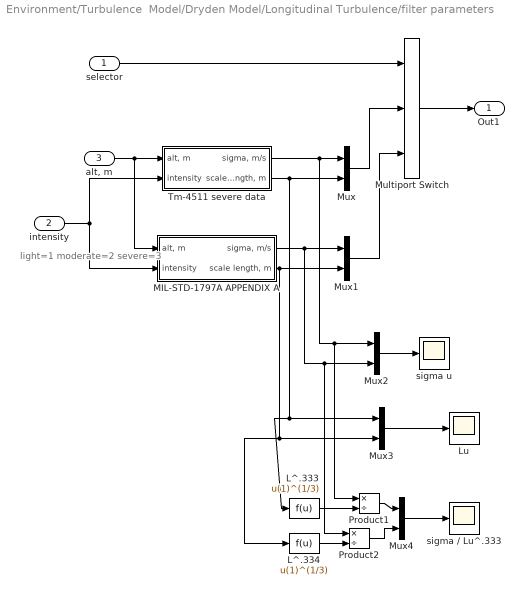
== system Environment/Turbulence  Model/Dryden Model/Longitudinal Turbulence/filter parameters ==
  note: light=1
      | moderate=2
      | severe=3
  selector : Inport
  intensity : Inport  Port=2
  "alt, m" : Inport  Port=3
  L^.333 : Fcn  Expr=u(1)^(1/3)
  L^.334 : Fcn  Expr=u(1)^(1/3)
  Lu : Scope
  "MIL-STD-1797A APPENDIX A " : Subsystem
  Multiport Switch : MultiPortSwitch  Inputs=2
  Mux{,1..4} (5 alike) : Mux  Inputs=2
  Product1 : Product  Inputs=*/  InputSameDT=on  SaturateOnIntegerOverflow=on  OutDataTypeStr=Inherit: Same as first input
  Product2 : Product  Inputs=*/  InputSameDT=on  SaturateOnIntegerOverflow=on  OutDataTypeStr=Inherit: Same as first input
  Tm-4511 severe data : Subsystem
  sigma / Lu^.333 : Scope
      settings: ActiveDisplayYMinimum=0  ActiveDisplayYMaximum=60
  sigma u : Scope
      settings: ActiveDisplayYMinimum=2  ActiveDisplayYMaximum=5.75
  Out1 : Outport
  wires:
  L^.334/1 -> Product2/2
  L^.333/1 -> Product1/2
  Product1/1 -> Mux4/1
  Product2/1 -> Mux4/2
  Mux4/1 -> sigma / Lu^.333/1
  "MIL-STD-1797A APPENDIX A "/2("scale length, m") -> L^.334/1, Mux3/2, Mux1/2
  Tm-4511 severe data/2("scale length, m") -> L^.333/1, Mux3/1, Mux/2
  "MIL-STD-1797A APPENDIX A "/1("sigma, m/s") -> Product2/1, Mux2/2, Mux1/1
  Mux2/1 -> sigma u/1
  Mux3/1 -> Lu/1
  intensity/1 -> Tm-4511 severe data/2(intensity), "MIL-STD-1797A APPENDIX A "/2(intensity)
  "alt, m"/1 -> "MIL-STD-1797A APPENDIX A "/1("alt, m"), Tm-4511 severe data/1("alt, m")
  Mux1/1 -> Multiport Switch/3
  Mux/1 -> Multiport Switch/2
  Tm-4511 severe data/1("sigma, m/s") -> Mux/1, Product1/1, Mux2/1
  Multiport Switch/1 -> Out1/1
  selector/1 -> Multiport Switch/1

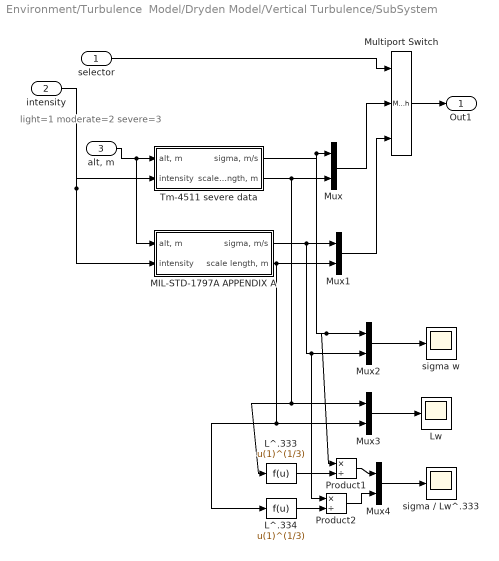
== system Environment/Turbulence  Model/Dryden Model/Vertical Turbulence/SubSystem ==
  note: light=1
      | moderate=2
      | severe=3
  selector : Inport
  "intensity " : Inport  Port=2
  "alt, m" : Inport  Port=3
  L^.333 : Fcn  Expr=u(1)^(1/3)
  L^.334 : Fcn  Expr=u(1)^(1/3)
  Lw : Scope
  "MIL-STD-1797A APPENDIX A " : Subsystem
  Multiport Switch : MultiPortSwitch  Inputs=2
  Mux{,1..4} (5 alike) : Mux  Inputs=2
  Product1 : Product  Inputs=*/  InputSameDT=on  SaturateOnIntegerOverflow=on  OutDataTypeStr=Inherit: Same as first input
  Product2 : Product  Inputs=*/  InputSameDT=on  SaturateOnIntegerOverflow=on  OutDataTypeStr=Inherit: Same as first input
  Tm-4511 severe data : Subsystem
  sigma / Lw^.333 : Scope
  sigma w : Scope
      settings: ActiveDisplayYMinimum=0.75  ActiveDisplayYMaximum=5.75
  Out1 : Outport
  wires:
  L^.334/1 -> Product2/2
  L^.333/1 -> Product1/2
  Product1/1 -> Mux4/1
  Product2/1 -> Mux4/2
  Mux4/1 -> sigma / Lw^.333/1
  Mux2/1 -> sigma w/1
  Mux3/1 -> Lw/1
  "MIL-STD-1797A APPENDIX A "/2("scale length, m") -> L^.334/1, Mux3/2, Mux1/2
  Tm-4511 severe data/2("scale length, m") -> L^.333/1, Mux3/1, Mux/2
  "MIL-STD-1797A APPENDIX A "/1("sigma, m/s") -> Product2/1, Mux2/2, Mux1/1
  Mux1/1 -> Multiport Switch/3
  Mux/1 -> Multiport Switch/2
  "intensity "/1 -> Tm-4511 severe data/2(intensity), "MIL-STD-1797A APPENDIX A "/2(intensity)
  "alt, m"/1 -> "MIL-STD-1797A APPENDIX A "/1("alt, m"), Tm-4511 severe data/1("alt, m")
  Tm-4511 severe data/1("sigma, m/s") -> Product1/1, Mux2/1, Mux/1
  Multiport Switch/1 -> Out1/1
  selector/1 -> Multiport Switch/1

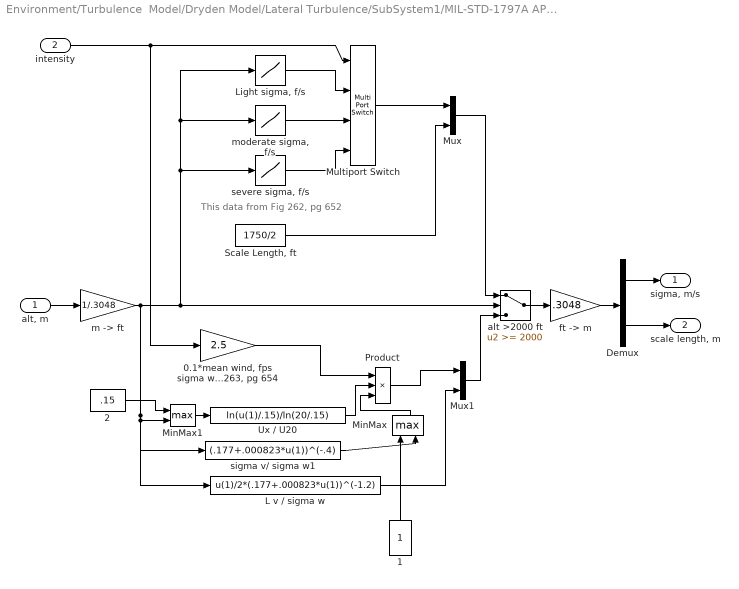
== system Environment/Turbulence  Model/Dryden Model/Lateral Turbulence/SubSystem1/MIL-STD-1797A APPENDIX A  ==
  note: This data from Fig 262, pg 652
  "alt, m" : Inport
  intensity : Inport  Port=2
  "0.1*mean wind, fps sigma w = to 2.5f/s * intensity Fig 263, pg 654" : Gain  Gain=2.5  SaturateOnIntegerOverflow=on  OutDataTypeStr=Inherit: Same as input  ParamDataTypeStr=Inherit: Same as input
  1 : Constant
  2 : Constant  Value=.15
  Demux : Demux  Outputs=2
      settings: DisplayOption=none
  L v / sigma w : Fcn  Expr=u(1)/2*(.177+.000823*u(1))^(-1.2)
  "Light sigma, f/s" : Lookup  InputValues=[2000 9000 18000 100000]  Table=[5 5 3 3]
  MinMax : MinMax  Function=max  Inputs=2  InputSameDT=on  SaturateOnIntegerOverflow=on
  MinMax1 : MinMax  Function=max  Inputs=2  InputSameDT=on  SaturateOnIntegerOverflow=on
  Multiport Switch : MultiPortSwitch
  Mux : Mux  Inputs=2
  Mux1 : Mux  Inputs=2
  Product : Product  Inputs=3  InputSameDT=on  SaturateOnIntegerOverflow=on  OutDataTypeStr=Inherit: Same as first input
  "Scale Length, ft" : Constant  Value=1750/2
  Ux / U20 : Fcn  Expr=ln(u(1)/.15)/ln(20/.15)
  alt >2000 ft : Switch  Threshold=2000
  "ft -> m" : Gain  Gain=.3048  SaturateOnIntegerOverflow=on  OutDataTypeStr=Inherit: Same as input  ParamDataTypeStr=Inherit: Same as input
  "m -> ft" : Gain  Gain=1/.3048  SaturateOnIntegerOverflow=on  OutDataTypeStr=Inherit: Same as input  ParamDataTypeStr=Inherit: Same as input
  "moderate sigma, f/s" : Lookup  InputValues=[2000 12000 44000 100000]  Table=[10 10 3 3]
  "severe sigma, f/s" : Lookup  InputValues=[2000 5000 22000 80000 100000]  Table=[15.5 21.5 21.5 3 3]
  sigma v/ sigma w1 : Fcn  Expr=(.177+.000823*u(1))^(-.4)
  "sigma, m/s" : Outport
  "scale length, m" : Outport  Port=2
  wires:
  Ux / U20/1 -> Product/2
  MinMax1/1 -> Ux / U20/1
  2/1 -> MinMax1/1
  "0.1*mean wind, fps sigma w = to 2.5f/s * intensity Fig 263, pg 654"/1 -> Product/1
  1/1 -> MinMax/1
  "ft -> m"/1 -> Demux/1
  alt >2000 ft/1 -> "ft -> m"/1
  Demux/1 -> "sigma, m/s"/1
  Demux/2 -> "scale length, m"/1
  L v / sigma w/1 -> Mux1/2
  Mux1/1 -> alt >2000 ft/3
  "m -> ft"/1 -> MinMax1/2, L v / sigma w/1, sigma v/ sigma w1/1, "moderate sigma, f/s"/1, "Light sigma, f/s"/1, "severe sigma, f/s"/1, alt >2000 ft/2
  "Scale Length, ft"/1 -> Mux/2
  intensity/1 -> "0.1*mean wind, fps sigma w = to 2.5f/s * intensity Fig 263, pg 654"/1, Multiport Switch/1
  Mux/1 -> alt >2000 ft/1
  Multiport Switch/1 -> Mux/1
  "alt, m"/1 -> "m -> ft"/1
  "severe sigma, f/s"/1 -> Multiport Switch/4
  "moderate sigma, f/s"/1 -> Multiport Switch/3
  "Light sigma, f/s"/1 -> Multiport Switch/2
  sigma v/ sigma w1/1 -> MinMax/2
  MinMax/1 -> Product/3
  Product/1 -> Mux1/1

== system Environment/Turbulence  Model/Dryden Model/Lateral Turbulence/SubSystem1/Tm-4511 severe data ==
  note: "Light" and "Moderate" sigmas are ZERO below 1km alt.
      | Table 2-79 does not define them.
  "alt, m" : Inport
  intensity : Inport  Port=2
  "Lateral sigma, m/s light TM-4511 Table 2-79" : Lookup  InputValues="[10 20 30 40 50 60 70 80 90 100 200 304.8 305 400  762 769 1000 2000 4000 6000 8000 10000 12000 14000 16000]"  Table="[0   0   0   0   0   0   0   0   0    0    0    0   0   0   0   0   .17  .17  .2   .21   .22   .22   .25   .26   .24   ]"
  "Lateral sigma, m/s moderate TM-4511 Table 2-79" : Lookup  InputValues="[10 20 30 40 50 60 70 80 90 100 200 304.8 305 400  762 769 1000 2000 4000 6000 8000 10000 12000 14000 16000]"  Table="[0   0  0    0    0   0  0  0   0   0     0    0      0     0      0    0  1.65  1.65 2.04 2.13 2.15 2.23 2.47 2.62 2.44]"
  "Lateral sigma, m/s severe TM-4511 Table 2-79" : Lookup  InputValues=[10 20 30 40 50 60 70 80 90 100 200 304.8 305 400 762 769 1000 2000 4000 6000 8000 10000 12000 14000 16000]  Table=[1.67 1.98 2.2 2.36 2.49 2.61 2.71 2.81 2.89 2.97 3.53 3.95 4.37 4.39 4.39 5.7 5.7 5.8 6.24 7.16 7.59 7.72 7.89 6.93 5]  LookUpMeth=Interpolation-Use End Values
  "Lateral, Scale, m TM-4511 Table 2-79" : Lookup  InputValues=[0 10 20 30 40 50 60 70 80 90 100 200 304.8 305 762 769 900 1000 2000 4000 6000 8000 10000 12000 14000 16000]  Table=[11 11 19 28 35 42 49 56 63 69 75 134 190 300 300 533 533 832 902 1040 1040 1040 1230 1800 2820 3400]  LookUpMeth=Interpolation-Use End Values
  Multiport Switch : MultiPortSwitch
  "sigma, m/s" : Outport
  "scale length, m" : Outport  Port=2
  wires:
  intensity/1 -> Multiport Switch/1
  "Lateral sigma, m/s light TM-4511 Table 2-79"/1 -> Multiport Switch/2
  "Lateral sigma, m/s moderate TM-4511 Table 2-79"/1 -> Multiport Switch/3
  "Lateral sigma, m/s severe TM-4511 Table 2-79"/1 -> Multiport Switch/4
  Multiport Switch/1 -> "sigma, m/s"/1
  "Lateral, Scale, m TM-4511 Table 2-79"/1 -> "scale length, m"/1
  "alt, m"/1 -> "Lateral sigma, m/s light TM-4511 Table 2-79"/1, "Lateral sigma, m/s moderate TM-4511 Table 2-79"/1, "Lateral, Scale, m TM-4511 Table 2-79"/1, "Lateral sigma, m/s severe TM-4511 Table 2-79"/1

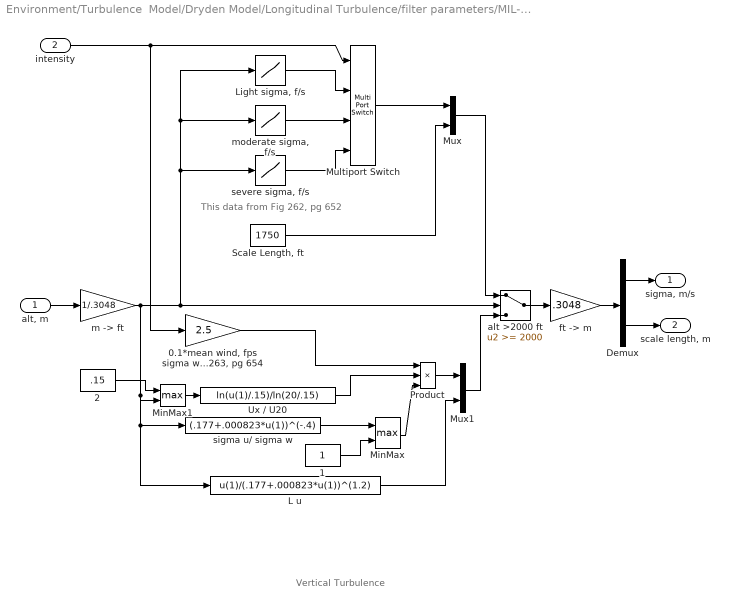
== system Environment/Turbulence  Model/Dryden Model/Longitudinal Turbulence/filter parameters/MIL-STD-1797A APPENDIX A  ==
  note: Vertical Turbulence
  note: This data from Fig 262, pg 652
  "alt, m" : Inport
  intensity : Inport  Port=2
  "0.1*mean wind, fps sigma w = to 2.5f/s * intensity Fig 263, pg 654" : Gain  Gain=2.5  SaturateOnIntegerOverflow=on  OutDataTypeStr=Inherit: Same as input  ParamDataTypeStr=Inherit: Same as input
  1 : Constant
  2 : Constant  Value=.15
  Demux : Demux  Outputs=2
      settings: DisplayOption=none
  "L u " : Fcn  Expr=u(1)/(.177+.000823*u(1))^(1.2)
  "Light sigma, f/s" : Lookup  InputValues=[2000 9000 18000 100000]  Table=[5 5 3 3]
  MinMax : MinMax  Function=max  Inputs=2  InputSameDT=on  SaturateOnIntegerOverflow=on
  MinMax1 : MinMax  Function=max  Inputs=2  InputSameDT=on  SaturateOnIntegerOverflow=on
  Multiport Switch : MultiPortSwitch
  Mux : Mux  Inputs=2
  Mux1 : Mux  Inputs=2
  Product : Product  Inputs=3  InputSameDT=on  SaturateOnIntegerOverflow=on  OutDataTypeStr=Inherit: Same as first input
  "Scale Length, ft" : Constant  Value=1750
  Ux / U20 : Fcn  Expr=ln(u(1)/.15)/ln(20/.15)
  alt >2000 ft : Switch  Threshold=2000
  "ft -> m" : Gain  Gain=.3048  SaturateOnIntegerOverflow=on  OutDataTypeStr=Inherit: Same as input  ParamDataTypeStr=Inherit: Same as input
  "m -> ft" : Gain  Gain=1/.3048  SaturateOnIntegerOverflow=on  OutDataTypeStr=Inherit: Same as input  ParamDataTypeStr=Inherit: Same as input
  "moderate sigma, f/s" : Lookup  InputValues=[2000 12000 44000 100000]  Table=[10 10 3 3]
  "severe sigma, f/s" : Lookup  InputValues=[2000 5000 22000 80000 100000]  Table=[15.5 21.5 21.5 3 3]
  sigma u/ sigma w : Fcn  Expr=(.177+.000823*u(1))^(-.4)
  "sigma, m/s" : Outport
  "scale length, m" : Outport  Port=2
  wires:
  Ux / U20/1 -> Product/2
  Product/1 -> Mux1/1
  MinMax/1 -> Product/3
  sigma u/ sigma w/1 -> MinMax/1
  1/1 -> MinMax/2
  MinMax1/1 -> Ux / U20/1
  2/1 -> MinMax1/1
  "0.1*mean wind, fps sigma w = to 2.5f/s * intensity Fig 263, pg 654"/1 -> Product/1
  "ft -> m"/1 -> Demux/1
  alt >2000 ft/1 -> "ft -> m"/1
  "L u "/1 -> Mux1/2
  Mux1/1 -> alt >2000 ft/3
  "m -> ft"/1 -> MinMax1/2, "L u "/1, sigma u/ sigma w/1, "moderate sigma, f/s"/1, "Light sigma, f/s"/1, "severe sigma, f/s"/1, alt >2000 ft/2
  Demux/1 -> "sigma, m/s"/1
  Demux/2 -> "scale length, m"/1
  "Scale Length, ft"/1 -> Mux/2
  intensity/1 -> "0.1*mean wind, fps sigma w = to 2.5f/s * intensity Fig 263, pg 654"/1, Multiport Switch/1
  Mux/1 -> alt >2000 ft/1
  Multiport Switch/1 -> Mux/1
  "alt, m"/1 -> "m -> ft"/1
  "severe sigma, f/s"/1 -> Multiport Switch/4
  "moderate sigma, f/s"/1 -> Multiport Switch/3
  "Light sigma, f/s"/1 -> Multiport Switch/2

== system Environment/Turbulence  Model/Dryden Model/Longitudinal Turbulence/filter parameters/Tm-4511 severe data ==
  note: "Light" and "Moderate" sigmas are ZERO below 1km alt.
      | Table 2-79 does not define them.
  "alt, m" : Inport
  intensity : Inport  Port=2
  "Longitudinal Scale, m TM-4511 Table 2-79" : Lookup  InputValues=[0 10 20 30 40 50 60 70 80 90 100 200 304.8 305 762 769 900 1000 2000 4000 6000 8000 10000 12000 14000 16000]  Table=[21 21 33 43 52 61 68 75 82 89 95 149 196 300 300 533 533 832 902 1040 1040 1040 1230 1800 2820 3400]
  "Longitudinal sigma, m/s light TM-4511 Table 2-79" : Lookup  InputValues="[10 20 30 40 50 60 70 80 90 100 200 304.8 305 400  762 769 1000 2000 4000 6000 8000 10000 12000 14000 16000]"  Table="[0   0   0   0   0   0   0   0   0    0    0    0   0   0   0   0   .17  .17  .2   .21   .22   .22   .25   .26   .24   ]"
  "Longitudinal sigma, m/s moderate TM-4511 Table 2-79" : Lookup  InputValues="[10 20 30 40 50 60 70 80 90 100 200 304.8 305 400  762 769 1000 2000 4000 6000 8000 10000 12000 14000 16000]"  Table="[0   0  0    0    0   0  0  0   0   0     0    0      0     0      0    0  1.65  1.65 2.04 2.13 2.15 2.23 2.47 2.62 2.44]"
  "Longitudinal sigma, m/s severe TM-4511 Table 2-79" : Lookup  InputValues="[10 20 30 40 50 60 70 80 90 100 200 304.8 305 400  762 769 1000 2000 4000 6000 8000 10000 12000 14000 16000]"  Table=[2.31 2.58 2.75 2.88 2.98 3.07 3.15 3.22 3.28 3.33 3.72 3.95 4.37 4.39 4.39 5.7 5.7 5.8 6.24 7.16 7.59 7.72 7.89 6.93 5]
  Multiport Switch : MultiPortSwitch
  "sigma, m/s" : Outport
  "scale length, m" : Outport  Port=2
  wires:
  intensity/1 -> Multiport Switch/1
  "Longitudinal sigma, m/s light TM-4511 Table 2-79"/1 -> Multiport Switch/2
  "Longitudinal sigma, m/s moderate TM-4511 Table 2-79"/1 -> Multiport Switch/3
  "Longitudinal sigma, m/s severe TM-4511 Table 2-79"/1 -> Multiport Switch/4
  Multiport Switch/1 -> "sigma, m/s"/1
  "Longitudinal Scale, m TM-4511 Table 2-79"/1 -> "scale length, m"/1
  "alt, m"/1 -> "Longitudinal sigma, m/s light TM-4511 Table 2-79"/1, "Longitudinal sigma, m/s moderate TM-4511 Table 2-79"/1, "Longitudinal Scale, m TM-4511 Table 2-79"/1, "Longitudinal sigma, m/s severe TM-4511 Table 2-79"/1

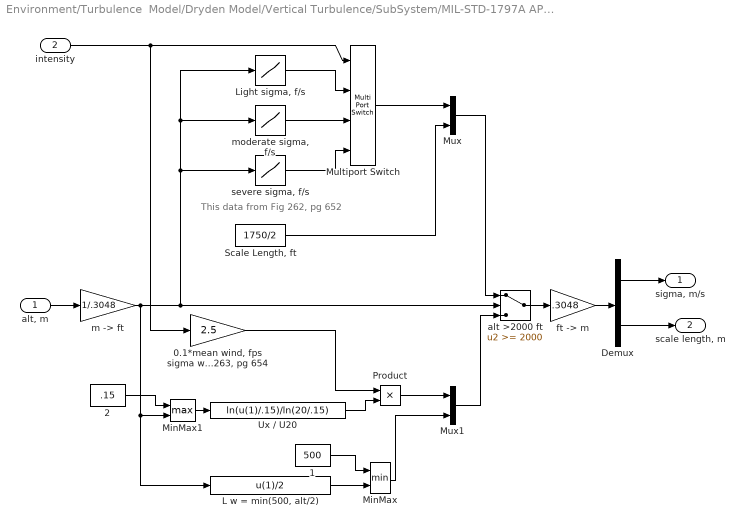
== system Environment/Turbulence  Model/Dryden Model/Vertical Turbulence/SubSystem/MIL-STD-1797A APPENDIX A  ==
  note: This data from Fig 262, pg 652
  "alt, m" : Inport
  intensity : Inport  Port=2
  "0.1*mean wind, fps sigma w = to 2.5f/s * intensity Fig 263, pg 654" : Gain  Gain=2.5  SaturateOnIntegerOverflow=on  OutDataTypeStr=Inherit: Same as input  ParamDataTypeStr=Inherit: Same as input
  1 : Constant  Value=500
  2 : Constant  Value=.15
  Demux : Demux  Outputs=2
      settings: DisplayOption=none
  "L w = min(500, alt/2)" : Fcn  Expr=u(1)/2
  "Light sigma, f/s" : Lookup  InputValues=[2000 9000 18000 100000]  Table=[5 5 3 3]
  MinMax : MinMax  Inputs=2  InputSameDT=on  SaturateOnIntegerOverflow=on
  MinMax1 : MinMax  Function=max  Inputs=2  InputSameDT=on  SaturateOnIntegerOverflow=on
  Multiport Switch : MultiPortSwitch
  Mux : Mux  Inputs=2
  Mux1 : Mux  Inputs=2
  Product : Product  InputSameDT=on  SaturateOnIntegerOverflow=on  OutDataTypeStr=Inherit: Same as first input
  "Scale Length, ft" : Constant  Value=1750/2
  Ux / U20 : Fcn  Expr=ln(u(1)/.15)/ln(20/.15)
  alt >2000 ft : Switch  Threshold=2000
  "ft -> m" : Gain  Gain=.3048  SaturateOnIntegerOverflow=on  OutDataTypeStr=Inherit: Same as input  ParamDataTypeStr=Inherit: Same as input
  "m -> ft" : Gain  Gain=1/.3048  SaturateOnIntegerOverflow=on  OutDataTypeStr=Inherit: Same as input  ParamDataTypeStr=Inherit: Same as input
  "moderate sigma, f/s" : Lookup  InputValues=[2000 12000 44000 100000]  Table=[10 10 3 3]
  "severe sigma, f/s" : Lookup  InputValues=[2000 5000 22000 80000 100000]  Table=[15.5 21.5 21.5 3 3]
  "sigma, m/s" : Outport
  "scale length, m" : Outport  Port=2
  wires:
  MinMax/1 -> Mux1/2
  Product/1 -> Mux1/1
  "0.1*mean wind, fps sigma w = to 2.5f/s * intensity Fig 263, pg 654"/1 -> Product/1
  Ux / U20/1 -> Product/2
  MinMax1/1 -> Ux / U20/1
  2/1 -> MinMax1/1
  "L w = min(500, alt/2)"/1 -> MinMax/2
  1/1 -> MinMax/1
  "ft -> m"/1 -> Demux/1
  alt >2000 ft/1 -> "ft -> m"/1
  Demux/1 -> "sigma, m/s"/1
  Demux/2 -> "scale length, m"/1
  Mux1/1 -> alt >2000 ft/3
  "m -> ft"/1 -> MinMax1/2, "L w = min(500, alt/2)"/1, "moderate sigma, f/s"/1, "Light sigma, f/s"/1, "severe sigma, f/s"/1, alt >2000 ft/2
  "Scale Length, ft"/1 -> Mux/2
  intensity/1 -> "0.1*mean wind, fps sigma w = to 2.5f/s * intensity Fig 263, pg 654"/1, Multiport Switch/1
  Mux/1 -> alt >2000 ft/1
  Multiport Switch/1 -> Mux/1
  "alt, m"/1 -> "m -> ft"/1
  "severe sigma, f/s"/1 -> Multiport Switch/4
  "moderate sigma, f/s"/1 -> Multiport Switch/3
  "Light sigma, f/s"/1 -> Multiport Switch/2

== system Environment/Turbulence  Model/Dryden Model/Vertical Turbulence/SubSystem/Tm-4511 severe data ==
  note: "Light" and "Moderate" sigmas are ZERO below 1km alt.
      | Table 2-79 does not define them.
  "alt, m" : Inport
  intensity : Inport  Port=2
  Multiport Switch : MultiPortSwitch
  "Vertical sigma, m/s light TM-4511 Table 2-79" : Lookup  InputValues="[10 20 30 40 50 60 70 80 90 100 200 304.8 305 400  762 769 1000 2000 4000 6000 8000 10000 12000 14000 16000]"  Table="[0   0   0   0   0   0   0   0   0    0    0    0   0   0   0   0   .14  .14  .17   .17   .17   .17   .18   .19   .21   ]"
  "Vertical sigma, m/s moderate TM-4511 Table 2-79" : Lookup  InputValues="[10 20 30 40 50 60 70 80 90 100 200 304.8 305 400  762 769 1000 2000 4000 6000 8000 10000 12000 14000 16000]"  Table="[0   0  0    0    0   0  0  0   0   0     0    0      0     0      0    0  1.36  1.43 1.68 1.69 1.695 1.73 1.79 1.91 2.1]"
  "Vertical Scale, m TM-4511 Table 2-79" : Lookup  InputValues=[0 10 20 30 40 50 60 70 80 90 100 200 304.8 305 762 769 900 1000 2000 4000 6000 8000 10000 12000 14000 16000]  Table=[ 5 5 11 17 23 29 35 41 47 53 59 123 192 300 300 533 533 624 831 972 1010 980 1100 1540 2120 2600]
  "Vertical sigma, m/s severe TM-4511 Table 2-79" : Lookup  InputValues=[10 20 30 40 50 60 70 80 90 100 200 304.8 305 762 769 900 1000 2000 4000 6000 8000 10000 12000 14000 16000]  Table=[1.15 1.46 1.71 1.89 2.05 2.19 2.32 2.43 2.54 2.64 3.38 3.95 4.39 4.39 5.7 5.7 4.67 4.75 5.13 5.69 5.98 6 5.71 5.05 4.31]
  "sigma, m/s" : Outport
  "scale length, m" : Outport  Port=2
  wires:
  "Vertical sigma, m/s severe TM-4511 Table 2-79"/1 -> Multiport Switch/4
  intensity/1 -> Multiport Switch/1
  "Vertical sigma, m/s light TM-4511 Table 2-79"/1 -> Multiport Switch/2
  "Vertical sigma, m/s moderate TM-4511 Table 2-79"/1 -> Multiport Switch/3
  Multiport Switch/1 -> "sigma, m/s"/1
  "Vertical Scale, m TM-4511 Table 2-79"/1 -> "scale length, m"/1
  "alt, m"/1 -> "Vertical sigma, m/s light TM-4511 Table 2-79"/1, "Vertical sigma, m/s moderate TM-4511 Table 2-79"/1, "Vertical sigma, m/s severe TM-4511 Table 2-79"/1, "Vertical Scale, m TM-4511 Table 2-79"/1

== matlab function Environment/atmos76 ==
  data: z input; y output; dt input
function y = layer1atm(z,dt)
% Author: Kevin Cunningham          April 20, 1992    
% Modified: Dave Cox                Aug, 14, 2008

y=zeros(6,1);

%dt=0;  % Standard Temp forced.

%    --- constants from 1976 std. atmosphere
r     = 1716.55915670803;
gamma = 1.4;
g     = 32.17405;
re    = 20855531.5;
tsl   = 288.15 * 1.8;
psl   = 2116.22;
hsl   = 0.;
sldens = 0.0023769;                 % atmospheric density at sea level
slpr   = 2116.220;                  % sea level pressure, psf

%---------------------------------------------------------------------
%    conversion from metric lapse rate to english lapse rate
%    meters/0.3048 = ft
%    Kelvin * 1.8 = Rankine
rm2ft = 1000.0/0.3048;
conlapse = 1.8/rm2ft;

%  ---- convert geometric alt. to geopotential alt.
h     = (re*z)/(re+z);
 
%  ---- ensure we are in layer one (based on geopotential alt)
if (h > 11*rm2ft) % 11 km
  %fprintf(1,'Error, atmosphere model out of range %f, Limiting...\n',h);
  h=11*rm2ft;
end
if (h<0)
  %fprintf(1,'Error, atmosphere model out of range %f, Limiting...\n',h);
  h=0;
end

a1     = -6.5*conlapse;
t1     = tsl + a1*(h-hsl);
del1   = (t1/tsl)^(-g/r/a1);
p1     = del1 * psl;

%   ---- apply temperature increment from standard day*/
t1     = t1 + dt;

%   ---- calculate density from eqn. of state w/ corrected temp.*/
rho1   = p1 / (r * t1);
 
%   ---- calculate speed of sound w/ corrected temp.*/
c1     = sqrt(gamma * (r * t1));
 

% Calculate outputs
y(1) = rho1;
y(2) = p1;
y(3) = t1 / 1.8; % output temperature  in Kelvin
y(4) = c1;
y(5) = y(2) / slpr;         % pressure ratio
y(6) = sqrt(y(1)/sldens);   % SQUARE ROOT OF DENSITY RATIO
